simulink model "WT_DYNAMIC_MODEL"  (R2025a)
settings: Solver=ode4  StartTime=0.0  StopTime=11  FixedStep=0.05  RelTol=1e-3
settings Model: Creator=hero  LastModifiedBy=hero

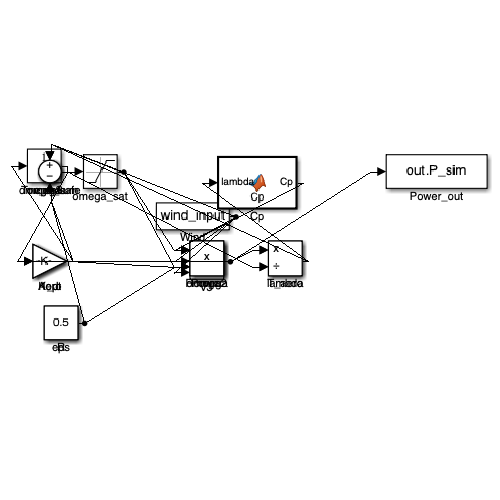
[thumbnail: Simulink's stored preview of the top-level diagram]
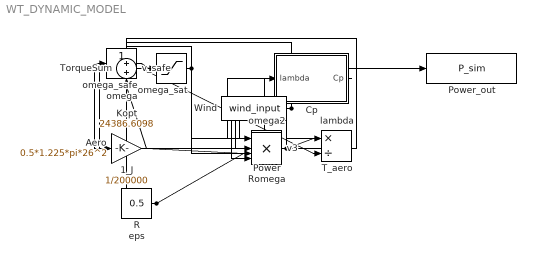
== system WT_DYNAMIC_MODEL ==
  1_J : Gain  Gain=1/200000
  Aero : Gain  Gain=0.5*1.225*pi*26^2
  Cp : MATLAB Function  TreatAsAtomicUnit=on
  Kopt : Gain  Gain=24386.6098
  Power : Product
  Power_out : ToWorkspace  VariableName=P_sim  SampleTime=-1
  R : Constant  Value=26
  Romega : Product
  T_aero : Product  Inputs=*/
  TorqueSum : Sum  Inputs=+-
  Wind : FromWorkspace  VariableName=wind_input
  eps : Constant  Value=0.5
  lambda : Product  Inputs=*/
  omega : Integrator  InitialCondition=6
  omega2 : Product
  omega_safe : Sum
  omega_sat : Saturate  UpperLimit=40  LowerLimit=0.5
  v3 : Product  Inputs=3
  v_safe : Sum
  wires:
  omega/1 -> omega_sat/1
  omega_sat/1 -> Romega/1, omega_safe/1, omega2/1, omega2/2
  R/1 -> Romega/2
  Wind/1 -> v_safe/1, v3/1, v3/2, v3/3
  eps/1 -> v_safe/2, omega_safe/2
  Romega/1 -> lambda/1
  v_safe/1 -> lambda/2
  lambda/1 -> Cp/1(lambda)
  v3/1 -> Aero/1
  Aero/1 -> Power/2
  Cp/1(Cp) -> Power/1
  Power/1 -> T_aero/1, Power_out/1
  omega_safe/1 -> T_aero/2
  omega2/1 -> Kopt/1
  T_aero/1 -> TorqueSum/1
  Kopt/1 -> TorqueSum/2
  TorqueSum/1 -> 1_J/1
  1_J/1 -> omega/1

== matlab function WT_DYNAMIC_MODEL/Cp ==
  data: lambda input; Cp output
function Cp = Cp(lambda)
lambda = max(lambda,0.1);
lambda_i = 1./(1./(lambda+0.08) - 0.035./(lambda.^3 + 1));
Cp = 0.22*((116./lambda_i)-5).*exp(-12.5./lambda_i);
Cp = max(0,min(0.45,Cp));
end
